simulink model "ros_controller"  (R2024a)
settings: Solver=FixedStepAuto  StartTime=0.0  StopTime=10.0  RelTol=1e-3
libraries: robotlib x5, simulink x2
settings Model: Creator=ianmi  LastModifiedBy=ianmi
settings OptimizationCC: EnhancedBackFolding=on  PassReuseOutputArgsAs=Individual arguments  ZeroExternalMemoryAtStartup=off  ZeroInternalMemoryAtStartup=off  MaxStackSize=64  OptimizeBlockOrder=speed  DifferentSizesBufferReuse=on  OptimizationCustomize=off  EfficientTunableParamExpr=on
settings DebuggingCC: ParameterTunabilityLossMsg=error
settings HardwareCC: ProdBitPerPointer=32  ProdBitPerSizeT=32  ProdBitPerPtrDiffT=32  ProdLargestAtomicFloat=None  ProdIntDivRoundTo=Undefined  ProdEndianess=Unspecified  ProdWordSize=32  ProdHWDeviceType=Generic->Unspecified (assume 32-bit Generic)  UseEmbeddedCoderFeatures=off
settings SFSimCC: MATLABDynamicMemAlloc=off
settings RTWCC: Description=Embedded Coder  SystemTargetFile=ert.tlc  HardwareBoard=Robot Operating System (ROS)  TLCOptions="-aInlineSetEventsForThisBaseRateFcn=TLC_FALSE -aSuppressMultiTaskScheduler=TLC_FALSE  -aRateBasedStepFcn=0"  GenCodeOnly=on  TemplateMakefile=ert_default_tmf  Toolchain=Catkin  TargetLang=C++
settings CodeAppCC: ForceParamTrailComments=on  IgnoreCustomStorageClasses=off  OperatorAnnotations=on  SimulinkDataObjDesc=on  SFDataObjDesc=on  InsertBlockDesc=on
settings ERTTargetCC: SupportNonInlinedSFcns=on

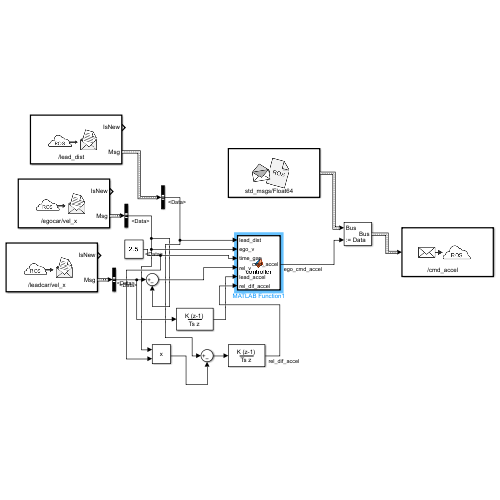
[thumbnail: Simulink's stored preview of the top-level diagram]
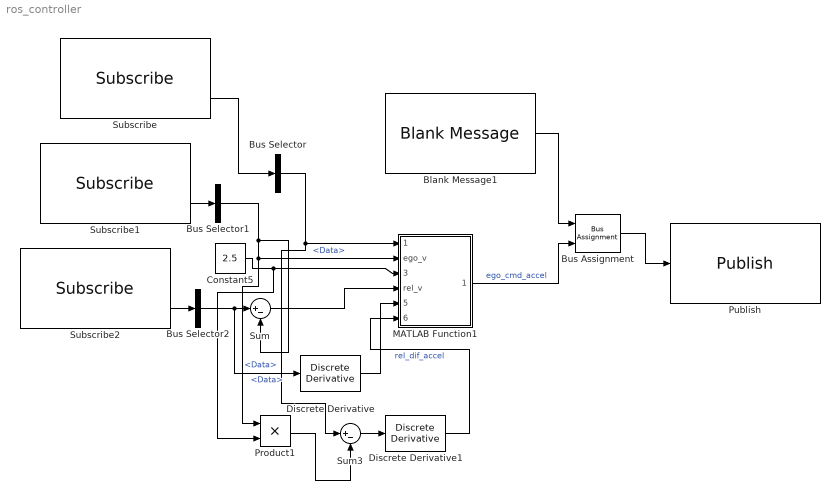
== system ros_controller ==
  Blank Message1 : robotlib/Blank Message  messageClass=Message  entityType=std_msgs/Float64  messageType=std_msgs/Float64  SampleTime=inf  legacyBusStruct=off
  Bus Assignment : BusAssignment  AssignedSignals=Data
  Bus Selector : BusSelector  OutputSignals=Data
  Bus Selector1 : BusSelector  OutputSignals=Data
  Bus Selector2 : BusSelector  OutputSignals=Data
  Constant5 : Constant  Value=2.5
  Discrete Derivative : simulink/Discrete/Discrete Derivative  gainval=1.0  ICPrevScaledInput=0.0  OutMin=[]  OutMax=[]  OutDataType=fixdt(1, 16)  OutScaling=2^-10  DoSatur=off
  Discrete Derivative1 : simulink/Discrete/Discrete Derivative  gainval=1.0  ICPrevScaledInput=0.0  OutMin=[]  OutMax=[]  OutDataType=fixdt(1, 16)  OutScaling=2^-10  DoSatur=off
  MATLAB Function1 : MATLAB Function  TreatAsAtomicUnit=on
  Product1 : Product
  Publish : robotlib/Publish  topicSource=Specify your own  topic=/cmd_accel  messageType=std_msgs/Float64  legacyBusStruct=off  messageQueueLength=1
  Subscribe : robotlib/Subscribe  topicSource=Specify your own  topic=/lead_dist  messageType=std_msgs/Float64  SampleTime=-1  legacyBusStruct=off  messageQueueLength=1
  Subscribe1 : robotlib/Subscribe  topicSource=Specify your own  topic=/egocar/vel_x  messageType=std_msgs/Float64  SampleTime=-1  legacyBusStruct=off  messageQueueLength=1
  Subscribe2 : robotlib/Subscribe  topicSource=Specify your own  topic=/leadcar/vel_x  messageType=std_msgs/Float64  SampleTime=-1  legacyBusStruct=off  messageQueueLength=1
  Sum : Sum  Inputs=|+-
  Sum3 : Sum  Inputs=|+-
  wires:
  Subscribe/2 -> Bus Selector/1
  Bus Selector/1 -> Sum3/1, MATLAB Function1/1(lead_dist)  "<Data>"
  Blank Message1/1 -> Bus Assignment/1
  Bus Assignment/1 -> Publish/1
  Subscribe1/2 -> Bus Selector1/1
  Constant5/1 -> Product1/2, MATLAB Function1/3(time_gap)
  Subscribe2/2 -> Bus Selector2/1
  Sum/1 -> MATLAB Function1/4(rel_v)
  Discrete Derivative/1 -> MATLAB Function1/5(lead_accel)
  Product1/1 -> Sum3/2
  Sum3/1 -> Discrete Derivative1/1
  Discrete Derivative1/1 -> MATLAB Function1/6(rel_dif_accel)  "rel_dif_accel"
  MATLAB Function1/1(cmd_accel) -> Bus Assignment/2  "ego_cmd_accel"
  Bus Selector1/1 -> Sum/2, Product1/1, MATLAB Function1/2(ego_v)  "<Data>"
  Bus Selector2/1 -> Discrete Derivative/1, Sum/1  "<Data>"

== matlab function ros_controller/MATLAB Function1 ==
  data: lead_dist input; ego_v input; time_gap input; rel_v input; cmd_accel output; lead_accel input; rel_dif_accel input
function cmd_accel = controller(lead_dist, ego_v, time_gap, rel_v, lead_accel, rel_dif_accel)

force = 0.4

alpha = 0.4
beta = 1
gamma = 0.2
delta = 0.1

cmd_accel = alpha * (-ego_v * time_gap + lead_dist)
cmd_accel = cmd_accel + beta * lead_accel
cmd_accel = cmd_accel + gamma * rel_dif_accel

cmd_accel = cmd_accel * force
if cmd_accel > 1.5
        cmd_accel = 1.5;
elseif cmd_accel < -3 
        cmd_accel = -3;
end
